simulink model "HistoryJunction1_2018a"  (R2018a)
settings: Solver=VariableStepAuto  StartTime=0.0  StopTime=10.0  RelTol=1e-3
settings Model: Creator=apple  LastModifiedBy=apple
settings DataIOCC: ReturnWorkspaceOutputs=on
settings SFSimCC: SimUseLocalCustomCode=on
settings RTWCC: RTWUseLocalCustomCode=on

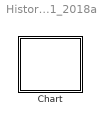
== system HistoryJunction1_2018a ==
  Chart : Stateflow chart  TreatAsAtomicUnit=on

== stateflow chart HistoryJunction1_2018a/Chart ==
  state B
    en:fprintf("Entry B");
    du:fprintf("During B");
    ex:fprintf("Exit B");
    (history)
    state B1
      en:fprintf("Entry B1");
    state B2
      en:fprintf("Entry B2");
    state B3
      en:fprintf("Entry B3");
    state B4
      en:fprintf("Entry B4");
    (default) -> B1
    B1 -> B2 : {x = x + 1;}
    B3 -> B1 : {x = x + 1;}
    B2 -> B4 : {x = x + 1;}
    B4 -> B3 : {x = x + 1;}
  state A
    en:fprintf("Entry A");
    du:fprintf("During A");
    ex:fprintf("Exit A");
  (default) -> A : {x= 0;}
  A -> B : E_one
  B -> A : [x>1]
  data: x local
  events: E_one local FUNCTION_CALL_EVENT
